simulink model "CrCtl_Governor"  (R2016b)
settings: configuration reference "CodeGenConfigSet" (kept outside this file)
values from neighbouring files (symbols this model uses):
  ACC_ZERO = fi(0,Acc_m_s2)    [init_CrCtl_Governor.m]
  CrCtl_facAcc2TrqCor_C = Calibration.Parameter    [init_CrCtl_Governor.m]
  CrCtl_facDecl2TrqCor_C = Calibration.Parameter    [init_CrCtl_Governor.m]
  CrCtl_facPT11_C = Calibration.Parameter    [init_CrCtl_Governor.m]
  CrCtl_facPT12_C = Calibration.Parameter    [init_CrCtl_Governor.m]
  CrCtl_facPT13_C = Calibration.Parameter    [init_CrCtl_Governor.m]
  CrCtl_facRmpSlpHiAcc_C = Calibration.Parameter    [init_CrCtl_Governor.m]
  CrCtl_facRmpSlpHiDecl_C = Calibration.Parameter    [init_CrCtl_Governor.m]
  CrCtl_facSlpConstRmpDwn_C = Calibration.Parameter    [init_CrCtl_Governor.m]
  CrCtl_facSlpConstRmpUp_C = Calibration.Parameter    [init_CrCtl_Governor.m]
  CrCtl_facSlpRmp1Sus_C = Calibration.Parameter    [init_CrCtl_Governor.m]
  CrCtl_facSlpRmp2Sus_C = Calibration.Parameter    [init_CrCtl_Governor.m]
  CrCtl_facTipDwnCor_CUR = Calibration.Parameter    [init_CrCtl_Governor.m]
  CrCtl_facTipDwnCor_CURX = Calibration.Parameter    [init_CrCtl_Governor.m]
  CrCtl_facTipUpCor_CUR = Calibration.Parameter    [init_CrCtl_Governor.m]
  CrCtl_facTipUpCor_CURX = Calibration.Parameter    [init_CrCtl_Governor.m]
  CrCtl_facTrqIncrSlpConstRmp_C = Calibration.Parameter    [init_CrCtl_Governor.m]
  CrCtl_facTrqIncrTimeConstRmp_C = Calibration.Parameter    [init_CrCtl_Governor.m]
  CrCtl_facTrqRedSlpConstRmp_C = Calibration.Parameter    [init_CrCtl_Governor.m]
  CrCtl_facTrqRedTimeConstRmp_C = Calibration.Parameter    [init_CrCtl_Governor.m]
  CrCtl_facTrqStrtAcc_C = Calibration.Parameter    [init_CrCtl_Governor.m]
  CrCtl_KiAcc1IWin_C = Calibration.Parameter    [init_CrCtl_Governor.m]
  CrCtl_KiAcc2IWin_C = Calibration.Parameter    [init_CrCtl_Governor.m]
  CrCtl_KiAcc3IWin_C = Calibration.Parameter    [init_CrCtl_Governor.m]
  CrCtl_KiCruise1IWin_C = Calibration.Parameter    [init_CrCtl_Governor.m]
  CrCtl_KiCruise2IWin_C = Calibration.Parameter    [init_CrCtl_Governor.m]
  CrCtl_KiCruise3IWin_C = Calibration.Parameter    [init_CrCtl_Governor.m]
  CrCtl_KiDecl1IWin_C = Calibration.Parameter    [init_CrCtl_Governor.m]
  CrCtl_KiDecl2IWin_C = Calibration.Parameter    [init_CrCtl_Governor.m]
  CrCtl_KiDecl3IWin_C = Calibration.Parameter    [init_CrCtl_Governor.m]
  CrCtl_KiNegAcc1IWin_C = Calibration.Parameter    [init_CrCtl_Governor.m]
  CrCtl_KiNegAcc2IWin_C = Calibration.Parameter    [init_CrCtl_Governor.m]
  CrCtl_KiNegAcc3IWin_C = Calibration.Parameter    [init_CrCtl_Governor.m]
  CrCtl_KiNegCruise1IWin_C = Calibration.Parameter    [init_CrCtl_Governor.m]
  CrCtl_KiNegCruise2IWin_C = Calibration.Parameter    [init_CrCtl_Governor.m]
  CrCtl_KiNegCruise3IWin_C = Calibration.Parameter    [init_CrCtl_Governor.m]
  CrCtl_KiNegDecl1IWin_C = Calibration.Parameter    [init_CrCtl_Governor.m]
  CrCtl_KiNegDecl2IWin_C = Calibration.Parameter    [init_CrCtl_Governor.m]
  CrCtl_KiNegDecl3IWin_C = Calibration.Parameter    [init_CrCtl_Governor.m]
  CrCtl_KiNegRes1IWin_C = Calibration.Parameter    [init_CrCtl_Governor.m]
  CrCtl_KiNegRes2IWin_C = Calibration.Parameter    [init_CrCtl_Governor.m]
  CrCtl_KiNegRes3IWin_C = Calibration.Parameter    [init_CrCtl_Governor.m]
  CrCtl_KiNegResCruise1IWin_C = Calibration.Parameter    [init_CrCtl_Governor.m]
  CrCtl_KiNegResCruise2IWin_C = Calibration.Parameter    [init_CrCtl_Governor.m]
  CrCtl_KiNegResCruise3IWin_C = Calibration.Parameter    [init_CrCtl_Governor.m]
  CrCtl_KiPosAcc1IWin_C = Calibration.Parameter    [init_CrCtl_Governor.m]
  CrCtl_KiPosAcc2IWin_C = Calibration.Parameter    [init_CrCtl_Governor.m]
  CrCtl_KiPosAcc3IWin_C = Calibration.Parameter    [init_CrCtl_Governor.m]
  CrCtl_KiPosCruise1IWin_C = Calibration.Parameter    [init_CrCtl_Governor.m]
  CrCtl_KiPosCruise2IWin_C = Calibration.Parameter    [init_CrCtl_Governor.m]
  CrCtl_KiPosCruise3IWin_C = Calibration.Parameter    [init_CrCtl_Governor.m]
  CrCtl_KiPosDecl1IWin_C = Calibration.Parameter    [init_CrCtl_Governor.m]
  CrCtl_KiPosDecl2IWin_C = Calibration.Parameter    [init_CrCtl_Governor.m]
  CrCtl_KiPosDecl3IWin_C = Calibration.Parameter    [init_CrCtl_Governor.m]
  CrCtl_KiPosRes1IWin_C = Calibration.Parameter    [init_CrCtl_Governor.m]
  CrCtl_KiPosRes3IWin_C = Calibration.Parameter    [init_CrCtl_Governor.m]
  CrCtl_KiPosResCruise1IWin_C = Calibration.Parameter    [init_CrCtl_Governor.m]
  CrCtl_KiPosResCruise2IWin_C = Calibration.Parameter    [init_CrCtl_Governor.m]
  CrCtl_KiPosResCruise3IWin_C = Calibration.Parameter    [init_CrCtl_Governor.m]
  CrCtl_KiRes1IWin_C = Calibration.Parameter    [init_CrCtl_Governor.m]
  CrCtl_KiRes2IWin_C = Calibration.Parameter    [init_CrCtl_Governor.m]
  CrCtl_KiRes3IWin_C = Calibration.Parameter    [init_CrCtl_Governor.m]
  CrCtl_KiResCruise1IWin_C = Calibration.Parameter    [init_CrCtl_Governor.m]
  CrCtl_KiResCruise2IWin_C = Calibration.Parameter    [init_CrCtl_Governor.m]
  CrCtl_KiResCruise3IWin_C = Calibration.Parameter    [init_CrCtl_Governor.m]
  CrCtl_KpAcc1PWin_C = Calibration.Parameter    [init_CrCtl_Governor.m]
  CrCtl_KpAcc2PWin_C = Calibration.Parameter    [init_CrCtl_Governor.m]
  CrCtl_KpAcc3PWin_C = Calibration.Parameter    [init_CrCtl_Governor.m]
  CrCtl_KpCruise1PWin_C = Calibration.Parameter    [init_CrCtl_Governor.m]
  CrCtl_KpCruise2PWin_C = Calibration.Parameter    [init_CrCtl_Governor.m]
  CrCtl_KpCruise3PWin_C = Calibration.Parameter    [init_CrCtl_Governor.m]
  CrCtl_KpDecl1PWin_C = Calibration.Parameter    [init_CrCtl_Governor.m]
  CrCtl_KpDecl2PWin_C = Calibration.Parameter    [init_CrCtl_Governor.m]
  CrCtl_KpDecl3PWin_C = Calibration.Parameter    [init_CrCtl_Governor.m]
  CrCtl_KpNegAcc1PWin_C = Calibration.Parameter    [init_CrCtl_Governor.m]
  CrCtl_KpNegAcc2PWin_C = Calibration.Parameter    [init_CrCtl_Governor.m]
  CrCtl_KpNegAcc3PWin_C = Calibration.Parameter    [init_CrCtl_Governor.m]
  CrCtl_KpNegCruise1PWin_C = Calibration.Parameter    [init_CrCtl_Governor.m]
  CrCtl_KpNegCruise2PWin_C = Calibration.Parameter    [init_CrCtl_Governor.m]
  CrCtl_KpNegCruise3PWin_C = Calibration.Parameter    [init_CrCtl_Governor.m]
  CrCtl_KpNegDecl1PWin_C = Calibration.Parameter    [init_CrCtl_Governor.m]
  CrCtl_KpNegDecl2PWin_C = Calibration.Parameter    [init_CrCtl_Governor.m]
  CrCtl_KpNegDecl3PWin_C = Calibration.Parameter    [init_CrCtl_Governor.m]
  CrCtl_KpNegRes1PWin_C = Calibration.Parameter    [init_CrCtl_Governor.m]
  CrCtl_KpNegRes2PWin_C = Calibration.Parameter    [init_CrCtl_Governor.m]
  CrCtl_KpNegRes3PWin_C = Calibration.Parameter    [init_CrCtl_Governor.m]
  CrCtl_KpNegResCruise1PWin_C = Calibration.Parameter    [init_CrCtl_Governor.m]
  CrCtl_KpNegResCruise2PWin_C = Calibration.Parameter    [init_CrCtl_Governor.m]
  CrCtl_KpNegResCruise3PWin_C = Calibration.Parameter    [init_CrCtl_Governor.m]
  CrCtl_KpPosAcc1PWin_C = Calibration.Parameter    [init_CrCtl_Governor.m]
  CrCtl_KpPosAcc2PWin_C = Calibration.Parameter    [init_CrCtl_Governor.m]
  CrCtl_KpPosAcc3PWin_C = Calibration.Parameter    [init_CrCtl_Governor.m]
  CrCtl_KpPosCruise1PWin_C = Calibration.Parameter    [init_CrCtl_Governor.m]
  CrCtl_KpPosCruise2PWin_C = Calibration.Parameter    [init_CrCtl_Governor.m]
  CrCtl_KpPosCruise3PWin_C = Calibration.Parameter    [init_CrCtl_Governor.m]
  CrCtl_KpPosDecl1PWin_C = Calibration.Parameter    [init_CrCtl_Governor.m]
  CrCtl_KpPosDecl2PWin_C = Calibration.Parameter    [init_CrCtl_Governor.m]
  CrCtl_KpPosDecl3PWin_C = Calibration.Parameter    [init_CrCtl_Governor.m]
  CrCtl_KpPosRes1PWin_C = Calibration.Parameter    [init_CrCtl_Governor.m]
  CrCtl_KpPosRes2PWin_C = Calibration.Parameter    [init_CrCtl_Governor.m]
  CrCtl_KpPosRes3PWin_C = Calibration.Parameter    [init_CrCtl_Governor.m]
  CrCtl_KpPosResCruise1PWin_C = Calibration.Parameter    [init_CrCtl_Governor.m]
  CrCtl_KpPosResCruise2PWin_C = Calibration.Parameter    [init_CrCtl_Governor.m]
  CrCtl_KpPosResCruise3PWin_C = Calibration.Parameter    [init_CrCtl_Governor.m]
  CrCtl_KpRes1PWin_C = Calibration.Parameter    [init_CrCtl_Governor.m]
  CrCtl_KpRes2PWin_C = Calibration.Parameter    [init_CrCtl_Governor.m]
  CrCtl_KpRes3PWin_C = Calibration.Parameter    [init_CrCtl_Governor.m]
  CrCtl_KpResCruise1PWin_C = Calibration.Parameter    [init_CrCtl_Governor.m]
  CrCtl_KpResCruise2PWin_C = Calibration.Parameter    [init_CrCtl_Governor.m]
  CrCtl_KpResCruise3PWin_C = Calibration.Parameter    [init_CrCtl_Governor.m]
  CrCtl_numParSelThres1_C = Calibration.Parameter    [init_CrCtl_Governor.m]
  CrCtl_numParSelThres2_C = Calibration.Parameter    [init_CrCtl_Governor.m]
  CrCtl_swtBrkMode_C = Calibration.Parameter    [init_CrCtl_Governor.m]
  CrCtl_swtILimWithP_C = Calibration.Parameter    [init_CrCtl_Governor.m]
  CrCtl_swtOvrRdeFrzInteg_C = Calibration.Parameter    [init_CrCtl_Governor.m]
  CrCtl_swtParSelHysBrk_C = Calibration.Parameter    [init_CrCtl_Governor.m]
  CrCtl_swtPT1EngBrk_C = Calibration.Parameter    [init_CrCtl_Governor.m]
  CrCtl_swtSusRmpInit_C = Calibration.Parameter    [init_CrCtl_Governor.m]
  CrCtl_swtSusRmpStp_C = Calibration.Parameter    [init_CrCtl_Governor.m]
  CrCtl_swtTipUpDwnGvnrStrtVal_C = Calibration.Parameter    [init_CrCtl_Governor.m]
  ... (+88 more)
undefined symbols (not defined in the file or in its folder): CrCtl_Governor_DT, CrCtl_stLck_conv, CrCtl_stOpFunc_conv, CrCtl_stShOff_conv, CrCtl_stSub_conv, CrCtl_stSuspRamp_conv, CruiseCtl_State_conv, EBrk_stPreSelMode_conv, WESDem_State_conv
libraries: CXLib x126, simulink x25
(part 4 of 6)

== system CrCtl_Governor/Cruise State/CRCTL_SUBGVNR/CrCtl_Suspend ==
  PT_trqWhlMinEng : Inport
  CrCtl_trqReqOld : Inport  Port=2
  AccPed_trqDes : Inport  Port=3
  CrCtl_trqLimAct : Inport  Port=4
  CrCtl_stSuspAct : Inport  Port=5
  Constant : Constant  Value=true
  Constant1 : Constant  Value=CrCtl_stSuspRamp_conv.CRCTL_SUSPENDENDRAMP
  Constant2 : Constant  Value=CrCtl_stSuspRamp_conv.CRCTL_SUSPENDRAMPDONE
  Constant3 : Constant  Value=CrCtl_stSuspRamp_conv.CRCTL_SUSPENDNOTACTIVE
  Constant4 : Constant  Value=CrCtl_stSuspRamp_conv.CRCTL_SUSPENDSTARTRAMP
  EdgeFalling : CXLib/EdgeFalling
  EdgeRising : CXLib/EdgeRising
  EdgeRising1 : CXLib/EdgeRising
  Logical Operator : Logic  Operator=NOT  AllPortsSameDT=off  OutDataTypeStr=boolean
  Subsystem : Subsystem
  Subsystem1 : Subsystem
  Switch{,1..3,5} (5 alike) : Switch  Criteria=u2 ~= 0
  Unit Delay : UnitDelay  SampleTime=-1
  CrCtl_stSuspRamp : Outport
  " CrCtl_trqReq" : Outport  Port=2
  wires:
  Subsystem/1(Out) -> Switch1/2, Subsystem1/5(In1)
  Subsystem/2(Out1) -> Switch5/1, Subsystem1/6(In2)
  PT_trqWhlMinEng/1 -> Subsystem/1(PT_trqWhlMinEng), Subsystem1/1(PT_trqWhlMinEng)
  CrCtl_trqReqOld/1 -> Subsystem/2(CrCtl_trqReqOld), Subsystem1/2(CrCtl_trqReqOld)
  CrCtl_trqLimAct/1 -> Subsystem1/4(CrCtl_trqLimAct)
  AccPed_trqDes/1 -> Subsystem1/3(AccPed_trqDes)
  Switch1/1 -> Switch/1
  Switch2/1 -> Switch/3
  Constant4/1 -> Switch1/1
  Constant2/1 -> Switch1/3
  Constant1/1 -> Switch2/1
  Constant3/1 -> Switch2/3
  Switch/1 -> CrCtl_stSuspRamp/1
  Subsystem1/1(Out1) -> Switch2/2
  Switch5/1 -> " CrCtl_trqReq"/1
  Subsystem1/2(Out2) -> Switch5/3
  Logical Operator/1 -> EdgeRising1/1
  EdgeRising/1 -> Subsystem/3(CrCtl_stSuspAct)
  EdgeRising1/1 -> Subsystem1/7(In3)
  CrCtl_stSuspAct/1 -> EdgeRising/1, EdgeFalling/1, Logical Operator/1, Subsystem/Enable, Switch/2, Switch5/2
  Constant/1 -> Switch3/1
  EdgeFalling/1 -> Switch3/2
  Switch3/1 -> Unit Delay/1, Subsystem1/Enable
  Unit Delay/1 -> Switch3/3

== system CrCtl_Governor/Cruise State/CRCTL_SUBGVNR/Governor ==
  CrCtl_trqLimAct : Inport
  CrCtl_trqMin : Inport  Port=2
  CrCtl_stGearRng_mp : Inport  Port=3
  CrCtl_vDesAct : Inport  Port=4
  stvHysEngBrkReq : Inport  Port=5
  GlbDa_vXFlt : Inport  Port=6
  stCrCtlOn : Inport  Port=7
  In1 : Inport  Port=8
  In2 : Inport  Port=9
  Enable : EnablePort
  Add1 : Sum  Inputs=+-
  Add2 : Sum  OutDataTypeStr=Trq_Nm
  Add3 : Sum  OutDataTypeStr=Trq_Nm
  Constant : Constant  Value=CrCtl_swtILimWithP_C
  Constant1 : Constant  Value=CrCtl_Governor_DT
  Constant2 : Constant  Value=1000  OutDataTypeStr=Inherit: Inherit via back propagation
  CrCtl_ARW : Subsystem
  I_S16 : CXLib/I_S16
  PT1 Filtered Torque : Subsystem
  P_S16 : CXLib/P_S16
  Parameter Selection for Ki : Subsystem
  Parameter Selection for Kp : Subsystem
  Product : Product  OutDataTypeStr=uint32
  Saturation_S16 : CXLib/Saturation_S16
  Switch : Switch  Criteria=u2 ~= 0
  Terminator : Terminator
  Unit Delay : UnitDelay  SampleTime=-1
  Unit Delay1 : UnitDelay  SampleTime=-1
  CrCtl_trqReq : Outport
  CrCtl_trqIWinOld_mp : Outport  Port=2  OutDataTypeStr=Trq_Nm
  CrCtl_trqReqPWin_mp : Outport  Port=3
  wires:
  CrCtl_vDesAct/1 -> Add1/1
  GlbDa_vXFlt/1 -> Add1/2
  Add1/1 -> PT1 Filtered Torque/2(vDiffCrCtl), I_S16/1, P_S16/1
  Add2/1 -> Add3/1
  PT1 Filtered Torque/1(CrCtl_trqDesvHys) -> Add3/2
  Add3/1 -> Saturation_S16/1
  CrCtl_trqMin/1 -> CrCtl_ARW/2(CrCtl_trqMin), Saturation_S16/2
  CrCtl_trqLimAct/1 -> CrCtl_ARW/3(CrCtl_trqLimAct), Saturation_S16/3
  Saturation_S16/2 -> Terminator/1
  Saturation_S16/1 -> CrCtl_trqReq/1
  Switch/1 -> CrCtl_ARW/5(CrCtl_trqReqIWin_mp), CrCtl_trqIWinOld_mp/1, Add2/2
  Constant/1 -> CrCtl_ARW/1(CrCtl_swtILimWithP_C)
  stvHysEngBrkReq/1 -> PT1 Filtered Torque/1(stvHysEngBrkReq)
  CrCtl_stGearRng_mp/1 -> Parameter Selection for Kp/1(CrCtl_stGearRng_mp), PT1 Filtered Torque/3(CrCtl_stGearRng_mp), Parameter Selection for Ki/1(CrCtl_stGearRng_mp)
  stCrCtlOn/1 -> PT1 Filtered Torque/4(stCrCtlOn)
  Parameter Selection for Kp/1(Out1) -> P_S16/2
  Parameter Selection for Kp/2(Out2) -> P_S16/3
  Parameter Selection for Kp/3(Out3) -> P_S16/4
  Parameter Selection for Kp/4(Out4) -> P_S16/5
  Parameter Selection for Kp/5(Out5) -> P_S16/6
  Parameter Selection for Ki/1(Out1) -> I_S16/3
  Parameter Selection for Ki/2(Out2) -> I_S16/4
  Parameter Selection for Ki/3(Out3) -> I_S16/5
  Parameter Selection for Ki/4(Out4) -> I_S16/6
  Parameter Selection for Ki/5(Out5) -> I_S16/7
  CrCtl_ARW/2(Limit) -> Unit Delay1/1
  CrCtl_ARW/1(CrCtl_stInit_mp) -> Unit Delay/1
  Product/1 -> I_S16/2
  Constant2/1 -> Product/2
  Constant1/1 -> Product/1
  I_S16/1 -> Switch/3
  Unit Delay1/1 -> Switch/1
  Unit Delay/1 -> Switch/2
  In1/1 -> I_S16/8
  In2/1 -> I_S16/9
  P_S16/1 -> CrCtl_trqReqPWin_mp/1, CrCtl_ARW/4(CrCtl_trqReqPWin_mp), Add2/1

== system CrCtl_Governor/Cruise State/CRCTL_SUBSTRTVAL/Parameter Selection for Kp ==
  CrCtl_stGearRng_mp : Inport
  Constant1 : Constant  Value=CrCtl_KpCruise2PWin_C
  Constant10 : Constant  Value=CrCtl_WinPosCruise1PWin_C
  Constant11 : Constant  Value=CrCtl_WinPosCruise2PWin_C
  Constant12 : Constant  Value=CrCtl_WinPosCruise2PWin_C
  Constant13 : Constant  Value=CrCtl_WinNegCruise1PWin_C
  Constant14 : Constant  Value=CrCtl_WinNegCruise2PWin_C
  Constant15 : Constant  Value=CrCtl_WinNegCruise3PWin_C
  Constant2 : Constant  Value=CrCtl_KpCruise3PWin_C
  Constant3 : Constant  Value=CrCtl_KpPosCruise1PWin_C
  Constant4 : Constant  Value=CrCtl_KpCruise1PWin_C
  Constant5 : Constant  Value=CrCtl_KpPosCruise2PWin_C
  Constant6 : Constant  Value=CrCtl_KpPosCruise3PWin_C
  Constant7 : Constant  Value=CrCtl_KpNegCruise1PWin_C
  Constant8 : Constant  Value=CrCtl_KpNegCruise2PWin_C
  Constant9 : Constant  Value=CrCtl_KpNegCruise3PWin_C
  Multiport Switch{,1..4} (5 alike) : MultiPortSwitch
  Out1 : Outport
  Out2 : Outport  Port=2
  Out3 : Outport  Port=3
  Out4 : Outport  Port=4
  Out5 : Outport  Port=5
  wires:
  CrCtl_stGearRng_mp/1 -> Multiport Switch4/1, Multiport Switch3/1, Multiport Switch2/1, Multiport Switch1/1, Multiport Switch/1
  Constant4/1 -> Multiport Switch/2
  Constant1/1 -> Multiport Switch/3
  Constant2/1 -> Multiport Switch/4
  Multiport Switch/1 -> Out1/1
  Constant3/1 -> Multiport Switch1/2
  Constant6/1 -> Multiport Switch1/4
  Constant5/1 -> Multiport Switch1/3
  Multiport Switch1/1 -> Out2/1
  Constant7/1 -> Multiport Switch2/2
  Constant9/1 -> Multiport Switch2/4
  Constant8/1 -> Multiport Switch2/3
  Constant10/1 -> Multiport Switch3/2
  Constant12/1 -> Multiport Switch3/4
  Constant11/1 -> Multiport Switch3/3
  Constant13/1 -> Multiport Switch4/2
  Constant15/1 -> Multiport Switch4/4
  Constant14/1 -> Multiport Switch4/3
  Multiport Switch2/1 -> Out3/1
  Multiport Switch3/1 -> Out4/1
  Multiport Switch4/1 -> Out5/1

== system CrCtl_Governor/Deceleration State/CRCTL_SUBRMP/CrCtl_OverRide ==
  CrCtl_trqLimAct : Inport
  CrCtl_trqMin : Inport  Port=2
  APP_r : Inport  Port=3
  AccPed_trqDes : Inport  Port=4
  CrCtl_vDes : Inport  Port=5
  GlbDa_vXFlt : Inport  Port=6
  CrCtl_trqReq : Inport  Port=7
  CrCtl_trqIWinOld_mp : Inport  Port=8
  Add : Sum
  Bit Clear : simulink/Logic and Bit Operations/Bit Clear  iBit=1
  Bit Clear7 : simulink/Logic and Bit Operations/Bit Clear  iBit=0
  Bit Set : simulink/Logic and Bit Operations/Bit Set  iBit=1
  Bit Set7 : simulink/Logic and Bit Operations/Bit Set  iBit=0
  Constant : Constant  Value=0
  Constant2 : Constant  Value=CrCtl_vCnclOverride_C
  Constant8 : Constant  Value=CrCtl_swtOvrRdeFrzInteg_C
  Logical Operator : Logic  AllPortsSameDT=off  OutDataTypeStr=boolean
  Logical Operator1 : Logic  AllPortsSameDT=off  OutDataTypeStr=boolean
  Relational Operator : RelationalOperator  Operator=>  OutDataTypeStr=boolean  RndMeth=Simplest
  Relational Operator1 : RelationalOperator  Operator=>  OutDataTypeStr=boolean  RndMeth=Simplest
  Relational Operator2 : RelationalOperator  Operator=<=  OutDataTypeStr=boolean  RndMeth=Simplest
  Relational Operator3 : RelationalOperator  Operator=<  OutDataTypeStr=boolean  RndMeth=Simplest
  Saturation_S16 : CXLib/Saturation_S16
  Switch : Switch  Criteria=u2 ~= 0
  Switch7 : Switch  Criteria=u2 ~= 0
  Switch8 : Switch  Criteria=u2 ~= 0
  Terminator1 : Terminator
  Unit Delay : UnitDelay  SampleTime=-1
  CrCtl_stIWin_mp : Outport
  CrCtl_trqReqIWin_mp : Outport  Port=2
  wires:
  APP_r/1 -> Relational Operator/1
  Constant/1 -> Relational Operator/2
  AccPed_trqDes/1 -> Relational Operator1/1, Relational Operator2/1
  Relational Operator/1 -> Logical Operator/1
  Relational Operator1/1 -> Logical Operator/2
  Logical Operator/1 -> Switch/2
  Relational Operator2/1 -> Logical Operator1/1
  Relational Operator3/1 -> Logical Operator1/2
  GlbDa_vXFlt/1 -> Relational Operator3/1
  CrCtl_vDes/1 -> Add/1
  Add/1 -> Relational Operator3/2
  Constant2/1 -> Add/2
  CrCtl_trqLimAct/1 -> Saturation_S16/3
  CrCtl_trqMin/1 -> Saturation_S16/2
  Bit Set/1 -> Switch/1
  Bit Clear/1 -> Switch/3
  Switch/1 -> Bit Clear7/1, Bit Set7/1
  Constant8/1 -> Switch7/2
  Bit Set7/1 -> Switch7/1
  Bit Clear7/1 -> Switch7/3
  Switch7/1 -> CrCtl_stIWin_mp/1, Unit Delay/1
  Unit Delay/1 -> Bit Set/1, Bit Clear/1
  CrCtl_trqReq/1 -> Saturation_S16/1
  Saturation_S16/1 -> Switch8/3, Relational Operator2/2, Relational Operator1/2
  Saturation_S16/2 -> Terminator1/1
  Logical Operator1/1 -> Switch8/2
  CrCtl_trqIWinOld_mp/1 -> Switch8/1
  Switch8/1 -> CrCtl_trqReqIWin_mp/1

== system CrCtl_Governor/Deceleration State/CRCTL_SUBRMP/CrCtl_Suspend ==
  PT_trqWhlMinEng : Inport
  CrCtl_trqReqOld : Inport  Port=2
  AccPed_trqDes : Inport  Port=3
  CrCtl_trqLimAct : Inport  Port=4
  CrCtl_stSuspAct : Inport  Port=5
  Constant : Constant  Value=true
  Constant1 : Constant  Value=CrCtl_stSuspRamp_conv.CRCTL_SUSPENDENDRAMP
  Constant2 : Constant  Value=CrCtl_stSuspRamp_conv.CRCTL_SUSPENDRAMPDONE
  Constant3 : Constant  Value=CrCtl_stSuspRamp_conv.CRCTL_SUSPENDNOTACTIVE
  Constant4 : Constant  Value=CrCtl_stSuspRamp_conv.CRCTL_SUSPENDSTARTRAMP
  EdgeFalling : CXLib/EdgeFalling
  EdgeRising : CXLib/EdgeRising
  EdgeRising1 : CXLib/EdgeRising
  Logical Operator : Logic  Operator=NOT  AllPortsSameDT=off  OutDataTypeStr=boolean
  Subsystem : Subsystem
  Subsystem1 : Subsystem
  Switch{,1..3,5} (5 alike) : Switch  Criteria=u2 ~= 0
  Unit Delay : UnitDelay  SampleTime=-1
  CrCtl_stSuspRamp : Outport
  " CrCtl_trqReq" : Outport  Port=2
  wires:
  Subsystem/1(Out) -> Switch1/2, Subsystem1/5(In1)
  Subsystem/2(Out1) -> Switch5/1, Subsystem1/6(In2)
  PT_trqWhlMinEng/1 -> Subsystem/1(PT_trqWhlMinEng), Subsystem1/1(PT_trqWhlMinEng)
  CrCtl_trqReqOld/1 -> Subsystem/2(CrCtl_trqReqOld), Subsystem1/2(CrCtl_trqReqOld)
  CrCtl_trqLimAct/1 -> Subsystem1/4(CrCtl_trqLimAct)
  AccPed_trqDes/1 -> Subsystem1/3(AccPed_trqDes)
  Switch1/1 -> Switch/1
  Switch2/1 -> Switch/3
  Constant4/1 -> Switch1/1
  Constant2/1 -> Switch1/3
  Constant1/1 -> Switch2/1
  Constant3/1 -> Switch2/3
  Switch/1 -> CrCtl_stSuspRamp/1
  Subsystem1/1(Out1) -> Switch2/2
  Switch5/1 -> " CrCtl_trqReq"/1
  Subsystem1/2(Out2) -> Switch5/3
  Logical Operator/1 -> EdgeRising1/1
  EdgeRising/1 -> Subsystem/3(CrCtl_stSuspAct)
  EdgeRising1/1 -> Subsystem1/7(In3)
  CrCtl_stSuspAct/1 -> EdgeRising/1, EdgeFalling/1, Logical Operator/1, Subsystem/Enable, Switch/2, Switch5/2
  Constant/1 -> Switch3/1
  EdgeFalling/1 -> Switch3/2
  Switch3/1 -> Unit Delay/1, Subsystem1/Enable
  Unit Delay/1 -> Switch3/3

== system CrCtl_Governor/Deceleration State/CRCTL_SUBRMP/Governor ==
  CrCtl_trqLimAct : Inport
  CrCtl_trqMin : Inport  Port=2
  CrCtl_stGearRng_mp : Inport  Port=3
  CrCtl_vDesAct : Inport  Port=4
  stvHysEngBrkReq : Inport  Port=5
  GlbDa_vXFlt : Inport  Port=6
  stCrCtlOn : Inport  Port=7
  In1 : Inport  Port=8
  In2 : Inport  Port=9
  Enable : EnablePort
  Add1 : Sum  Inputs=+-
  Add2 : Sum  OutDataTypeStr=Trq_Nm
  Add3 : Sum  OutDataTypeStr=Trq_Nm
  Constant : Constant  Value=CrCtl_swtILimWithP_C
  Constant1 : Constant  Value=CrCtl_Governor_DT
  Constant2 : Constant  Value=1000  OutDataTypeStr=Inherit: Inherit via back propagation
  CrCtl_ARW : Subsystem
  I_S16 : CXLib/I_S16
  PT1 Filtered Torque : Subsystem
  P_S16 : CXLib/P_S16
  Parameter Selection for Ki : Subsystem
  Parameter Selection for Kp : Subsystem
  Product : Product  OutDataTypeStr=uint32
  Saturation_S16 : CXLib/Saturation_S16
  Switch : Switch  Criteria=u2 ~= 0
  Terminator : Terminator
  Unit Delay : UnitDelay  SampleTime=-1
  Unit Delay1 : UnitDelay  SampleTime=-1
  CrCtl_trqReq : Outport
  CrCtl_trqIWinOld_mp : Outport  Port=2  OutDataTypeStr=Trq_Nm
  CrCtl_trqReqPWin_mp : Outport  Port=3
  wires:
  CrCtl_vDesAct/1 -> Add1/1
  GlbDa_vXFlt/1 -> Add1/2
  Add1/1 -> PT1 Filtered Torque/2(vDiffCrCtl), I_S16/1, P_S16/1
  Add2/1 -> Add3/1
  PT1 Filtered Torque/1(CrCtl_trqDesvHys) -> Add3/2
  Add3/1 -> Saturation_S16/1
  CrCtl_trqMin/1 -> CrCtl_ARW/2(CrCtl_trqMin), Saturation_S16/2
  CrCtl_trqLimAct/1 -> CrCtl_ARW/3(CrCtl_trqLimAct), Saturation_S16/3
  Saturation_S16/2 -> Terminator/1
  Saturation_S16/1 -> CrCtl_trqReq/1
  Switch/1 -> CrCtl_ARW/5(CrCtl_trqReqIWin_mp), CrCtl_trqIWinOld_mp/1, Add2/2
  Constant/1 -> CrCtl_ARW/1(CrCtl_swtILimWithP_C)
  stvHysEngBrkReq/1 -> PT1 Filtered Torque/1(stvHysEngBrkReq)
  CrCtl_stGearRng_mp/1 -> Parameter Selection for Kp/1(CrCtl_stGearRng_mp), Parameter Selection for Ki/1(CrCtl_stGearRng_mp), PT1 Filtered Torque/3(CrCtl_stGearRng_mp)
  stCrCtlOn/1 -> PT1 Filtered Torque/4(stCrCtlOn)
  Parameter Selection for Kp/1(Out1) -> P_S16/2
  Parameter Selection for Kp/2(Out2) -> P_S16/3
  Parameter Selection for Kp/3(Out3) -> P_S16/4
  Parameter Selection for Kp/4(Out4) -> P_S16/5
  Parameter Selection for Kp/5(Out5) -> P_S16/6
  Parameter Selection for Ki/1(Out1) -> I_S16/3
  Parameter Selection for Ki/2(Out2) -> I_S16/4
  Parameter Selection for Ki/3(Out3) -> I_S16/5
  Parameter Selection for Ki/4(Out4) -> I_S16/6
  Parameter Selection for Ki/5(Out5) -> I_S16/7
  CrCtl_ARW/2(Limit) -> Unit Delay1/1
  CrCtl_ARW/1(CrCtl_stInit_mp) -> Unit Delay/1
  Product/1 -> I_S16/2
  Constant2/1 -> Product/2
  Constant1/1 -> Product/1
  P_S16/1 -> CrCtl_trqReqPWin_mp/1, CrCtl_ARW/4(CrCtl_trqReqPWin_mp), Add2/1
  In1/1 -> I_S16/8
  In2/1 -> I_S16/9
  I_S16/1 -> Switch/3
  Unit Delay1/1 -> Switch/1
  Unit Delay/1 -> Switch/2

== system CrCtl_Governor/OFF State/CRCTL_SUBRMP/Immediate Shut off demanded ==
  PT_trqWhlMinEng : Inport
  Enable : EnablePort
  CrCtl_trqReq : Outport
  wires:
  PT_trqWhlMinEng/1 -> CrCtl_trqReq/1

== system CrCtl_Governor/OFF State/CRCTL_SUBRMP/Shut off by Slope Constant Ramp demanded ==
  PT_trqWhlMinEng : Inport
  CrCtl_trqReqOld : Inport  Port=2
  In1 : Inport  Port=3
  Enable : EnablePort
  Add : Sum
  Add1 : Sum  Inputs=+-
  Add2 : Sum  Inputs=+-
  Add3 : Sum  Inputs=+-
  Constant : Constant  Value=CrCtl_facTrqIncrSlpConstRmp_C
  Constant1 : Constant  Value=CrCtl_Governor_DT
  Constant2 : Constant  Value=CrCtl_facTrqRedSlpConstRmp_C
  Constant3 : Constant  Value=CrCtl_facSlpConstRmpUp_C
  Constant4 : Constant  Value=CrCtl_Governor_DT
  Constant5 : Constant  Value=CrCtl_facSlpConstRmpDwn_C
  Product : Product  OutDataTypeStr=Trq_Nm
  Product1 : Product  OutDataTypeStr=Trq_Nm
  RAMP_S16 : CXLib/RAMP_S16
  Relational Operator : RelationalOperator  Operator=>  OutDataTypeStr=boolean  RndMeth=Simplest
  Switch : Switch  Criteria=u2 ~= 0
  s2dt : CXLib/s2dt
  s2dt1 : CXLib/s2dt
  CrCtl_trqReq : Outport
  wires:
  s2dt/1 -> RAMP_S16/2
  Constant3/1 -> s2dt/1
  Constant4/1 -> s2dt/2
  Switch/1 -> RAMP_S16/5
  Constant1/1 -> s2dt1/2
  PT_trqWhlMinEng/1 -> RAMP_S16/1, Relational Operator/2, Add2/2, Add1/1
  Relational Operator/1 -> Switch/2
  CrCtl_trqReqOld/1 -> Add/1, Relational Operator/1, Add1/2, Add3/1, Add2/1
  Add1/1 -> Product/1
  Add2/1 -> Product1/2
  Constant/1 -> Product/2
  Constant2/1 -> Product1/1
  Product/1 -> Add/2
  Product1/1 -> Add3/2
  Add/1 -> Switch/3
  Add3/1 -> Switch/1
  s2dt1/1 -> RAMP_S16/3
  Constant5/1 -> s2dt1/1
  In1/1 -> RAMP_S16/4
  RAMP_S16/1 -> CrCtl_trqReq/1

== system CrCtl_Governor/OFF State/CRCTL_SUBRMP/Shut off by Time Constant Ramp demanded ==
  PT_trqWhlMinEng : Inport
  CrCtl_trqReqOld : Inport  Port=2
  In1 : Inport  Port=3
  Enable : EnablePort
  Abs : Abs
  Add : Sum
  Add1 : Sum  Inputs=+-
  Add2 : Sum  Inputs=+-
  Add3 : Sum  Inputs=+-
  Constant : Constant  Value=CrCtl_facTrqIncrTimeConstRmp_C
  Constant1 : Constant  Value=CrCtl_Governor_DT
  Constant2 : Constant  Value=CrCtl_facTrqRedTimeConstRmp_C
  Constant4 : Constant  Value=CrCtl_Governor_DT
  Constant6 : Constant  Value=CrCtl_tiShDwnTimeCnstRmp_C
  Divide : Product  Inputs=*/  OutDataTypeStr=Inherit: Inherit via back propagation
  Product : Product  OutDataTypeStr=Trq_Nm
  Product1 : Product  OutDataTypeStr=Trq_Nm
  RAMP_S16 : CXLib/RAMP_S16
  Relational Operator : RelationalOperator  Operator=>  OutDataTypeStr=boolean  RndMeth=Simplest
  Switch : Switch  Criteria=u2 ~= 0
  s2dt : CXLib/s2dt
  s2dt1 : CXLib/s2dt
  CrCtl_trqReq : Outport
  wires:
  PT_trqWhlMinEng/1 -> RAMP_S16/1, Add2/2, Add1/1, Relational Operator/2
  Relational Operator/1 -> Switch/2
  CrCtl_trqReqOld/1 -> Add2/1, Add3/1, Add1/2, Add/1, Relational Operator/1
  Add1/1 -> Abs/1, Product/1
  Add2/1 -> Product1/2
  Constant/1 -> Product/2
  Constant2/1 -> Product1/1
  Product/1 -> Add/2
  Product1/1 -> Add3/2
  Add/1 -> Switch/3
  Add3/1 -> Switch/1
  Divide/1 -> s2dt/1, s2dt1/1  "CrCtl_facShDwnTimeCnstRmp_mp"
  Constant4/1 -> s2dt/2
  Constant1/1 -> s2dt1/2
  s2dt1/1 -> RAMP_S16/3
  RAMP_S16/1 -> CrCtl_trqReq/1
  Abs/1 -> Divide/1
  Constant6/1 -> Divide/2
  In1/1 -> RAMP_S16/4
  Switch/1 -> RAMP_S16/5
  s2dt/1 -> RAMP_S16/2

== system CrCtl_Governor/Resume From Above/CRCTL_SUBRMP/CrCtl_OverRide ==
  CrCtl_trqLimAct : Inport
  CrCtl_trqMin : Inport  Port=2
  APP_r : Inport  Port=3
  AccPed_trqDes : Inport  Port=4
  CrCtl_vDes : Inport  Port=5
  GlbDa_vXFlt : Inport  Port=6
  CrCtl_trqReq : Inport  Port=7
  CrCtl_trqIWinOld_mp : Inport  Port=8
  Add : Sum
  Bit Clear : simulink/Logic and Bit Operations/Bit Clear  iBit=1
  Bit Clear7 : simulink/Logic and Bit Operations/Bit Clear  iBit=0
  Bit Set : simulink/Logic and Bit Operations/Bit Set  iBit=1
  Bit Set7 : simulink/Logic and Bit Operations/Bit Set  iBit=0
  Constant : Constant  Value=0
  Constant2 : Constant  Value=CrCtl_vCnclOverride_C
  Constant8 : Constant  Value=CrCtl_swtOvrRdeFrzInteg_C
  Logical Operator : Logic  AllPortsSameDT=off  OutDataTypeStr=boolean
  Logical Operator1 : Logic  AllPortsSameDT=off  OutDataTypeStr=boolean
  Relational Operator : RelationalOperator  Operator=>  OutDataTypeStr=boolean  RndMeth=Simplest
  Relational Operator1 : RelationalOperator  Operator=>  OutDataTypeStr=boolean  RndMeth=Simplest
  Relational Operator2 : RelationalOperator  Operator=<=  OutDataTypeStr=boolean  RndMeth=Simplest
  Relational Operator3 : RelationalOperator  Operator=<  OutDataTypeStr=boolean  RndMeth=Simplest
  Saturation_S16 : CXLib/Saturation_S16
  Switch : Switch  Criteria=u2 ~= 0
  Switch7 : Switch  Criteria=u2 ~= 0
  Switch8 : Switch  Criteria=u2 ~= 0
  Terminator1 : Terminator
  Unit Delay : UnitDelay  SampleTime=-1
  CrCtl_stIWin_mp : Outport
  CrCtl_trqReqIWin_mp : Outport  Port=2
  wires:
  APP_r/1 -> Relational Operator/1
  Constant/1 -> Relational Operator/2
  AccPed_trqDes/1 -> Relational Operator1/1, Relational Operator2/1
  Relational Operator/1 -> Logical Operator/1
  Relational Operator1/1 -> Logical Operator/2
  Logical Operator/1 -> Switch/2
  Relational Operator2/1 -> Logical Operator1/1
  Relational Operator3/1 -> Logical Operator1/2
  GlbDa_vXFlt/1 -> Relational Operator3/1
  CrCtl_vDes/1 -> Add/1
  Add/1 -> Relational Operator3/2
  Constant2/1 -> Add/2
  CrCtl_trqLimAct/1 -> Saturation_S16/3
  CrCtl_trqMin/1 -> Saturation_S16/2
  Bit Set/1 -> Switch/1
  Bit Clear/1 -> Switch/3
  Switch/1 -> Bit Clear7/1, Bit Set7/1
  Constant8/1 -> Switch7/2
  Bit Set7/1 -> Switch7/1
  Bit Clear7/1 -> Switch7/3
  Switch7/1 -> CrCtl_stIWin_mp/1, Unit Delay/1
  Unit Delay/1 -> Bit Set/1, Bit Clear/1
  CrCtl_trqReq/1 -> Saturation_S16/1
  Saturation_S16/1 -> Switch8/3, Relational Operator2/2, Relational Operator1/2
  Saturation_S16/2 -> Terminator1/1
  Logical Operator1/1 -> Switch8/2
  CrCtl_trqIWinOld_mp/1 -> Switch8/1
  Switch8/1 -> CrCtl_trqReqIWin_mp/1

== system CrCtl_Governor/Resume From Above/CRCTL_SUBRMP/CrCtl_Suspend ==
  PT_trqWhlMinEng : Inport
  CrCtl_trqReqOld : Inport  Port=2
  AccPed_trqDes : Inport  Port=3
  CrCtl_trqLimAct : Inport  Port=4
  CrCtl_stSuspAct : Inport  Port=5
  Constant : Constant  Value=true
  Constant1 : Constant  Value=CrCtl_stSuspRamp_conv.CRCTL_SUSPENDENDRAMP
  Constant2 : Constant  Value=CrCtl_stSuspRamp_conv.CRCTL_SUSPENDRAMPDONE
  Constant3 : Constant  Value=CrCtl_stSuspRamp_conv.CRCTL_SUSPENDNOTACTIVE
  Constant4 : Constant  Value=CrCtl_stSuspRamp_conv.CRCTL_SUSPENDSTARTRAMP
  EdgeFalling : CXLib/EdgeFalling
  EdgeRising : CXLib/EdgeRising
  EdgeRising1 : CXLib/EdgeRising
  Logical Operator : Logic  Operator=NOT  AllPortsSameDT=off  OutDataTypeStr=boolean
  Subsystem : Subsystem
  Subsystem1 : Subsystem
  Switch{,1..3,5} (5 alike) : Switch  Criteria=u2 ~= 0
  Unit Delay : UnitDelay  SampleTime=-1
  CrCtl_stSuspRamp : Outport
  " CrCtl_trqReq" : Outport  Port=2
  wires:
  Subsystem/1(Out) -> Switch1/2, Subsystem1/5(In1)
  Subsystem/2(Out1) -> Switch5/1, Subsystem1/6(In2)
  PT_trqWhlMinEng/1 -> Subsystem/1(PT_trqWhlMinEng), Subsystem1/1(PT_trqWhlMinEng)
  CrCtl_trqReqOld/1 -> Subsystem/2(CrCtl_trqReqOld), Subsystem1/2(CrCtl_trqReqOld)
  CrCtl_trqLimAct/1 -> Subsystem1/4(CrCtl_trqLimAct)
  AccPed_trqDes/1 -> Subsystem1/3(AccPed_trqDes)
  Switch1/1 -> Switch/1
  Switch2/1 -> Switch/3
  Constant4/1 -> Switch1/1
  Constant2/1 -> Switch1/3
  Constant1/1 -> Switch2/1
  Constant3/1 -> Switch2/3
  Switch/1 -> CrCtl_stSuspRamp/1
  Subsystem1/1(Out1) -> Switch2/2
  Switch5/1 -> " CrCtl_trqReq"/1
  Subsystem1/2(Out2) -> Switch5/3
  Logical Operator/1 -> EdgeRising1/1
  EdgeRising/1 -> Subsystem/3(CrCtl_stSuspAct)
  EdgeRising1/1 -> Subsystem1/7(In3)
  CrCtl_stSuspAct/1 -> EdgeRising/1, EdgeFalling/1, Logical Operator/1, Subsystem/Enable, Switch/2, Switch5/2
  Constant/1 -> Switch3/1
  EdgeFalling/1 -> Switch3/2
  Switch3/1 -> Unit Delay/1, Subsystem1/Enable
  Unit Delay/1 -> Switch3/3

== system CrCtl_Governor/Resume From Above/CRCTL_SUBRMP/Governor ==
  CrCtl_trqLimAct : Inport
  CrCtl_trqMin : Inport  Port=2
  CrCtl_stGearRng_mp : Inport  Port=3
  CrCtl_vDesAct : Inport  Port=4
  stvHysEngBrkReq : Inport  Port=5
  GlbDa_vXFlt : Inport  Port=6
  stCrCtlOn : Inport  Port=7
  In1 : Inport  Port=8
  In2 : Inport  Port=9
  Enable : EnablePort
  Add1 : Sum  Inputs=+-
  Add2 : Sum  OutDataTypeStr=Trq_Nm
  Add3 : Sum  OutDataTypeStr=Trq_Nm
  Constant : Constant  Value=CrCtl_swtILimWithP_C
  Constant1 : Constant  Value=CrCtl_Governor_DT
  Constant2 : Constant  Value=1000  OutDataTypeStr=Inherit: Inherit via back propagation
  CrCtl_ARW : Subsystem
  I_S16 : CXLib/I_S16
  PT1 Filtered Torque : Subsystem
  P_S16 : CXLib/P_S16
  Parameter Selection for Ki : Subsystem
  Parameter Selection for Kp : Subsystem
  Product : Product  OutDataTypeStr=uint32
  Saturation_S16 : CXLib/Saturation_S16
  Switch : Switch  Criteria=u2 ~= 0
  Terminator : Terminator
  Unit Delay : UnitDelay  SampleTime=-1
  Unit Delay1 : UnitDelay  SampleTime=-1
  CrCtl_trqReq : Outport
  CrCtl_trqIWinOld_mp : Outport  Port=2  OutDataTypeStr=Trq_Nm
  CrCtl_trqReqPWin_mp : Outport  Port=3
  wires:
  CrCtl_vDesAct/1 -> Add1/1
  GlbDa_vXFlt/1 -> Add1/2
  Add1/1 -> PT1 Filtered Torque/2(vDiffCrCtl), I_S16/1, P_S16/1
  Add2/1 -> Add3/1
  PT1 Filtered Torque/1(CrCtl_trqDesvHys) -> Add3/2
  Add3/1 -> Saturation_S16/1
  CrCtl_trqMin/1 -> CrCtl_ARW/2(CrCtl_trqMin), Saturation_S16/2
  CrCtl_trqLimAct/1 -> CrCtl_ARW/3(CrCtl_trqLimAct), Saturation_S16/3
  Saturation_S16/2 -> Terminator/1
  Saturation_S16/1 -> CrCtl_trqReq/1
  Switch/1 -> Add2/2, CrCtl_trqIWinOld_mp/1, CrCtl_ARW/5(CrCtl_trqReqIWin_mp)
  Constant/1 -> CrCtl_ARW/1(CrCtl_swtILimWithP_C)
  stvHysEngBrkReq/1 -> PT1 Filtered Torque/1(stvHysEngBrkReq)
  CrCtl_stGearRng_mp/1 -> Parameter Selection for Kp/1(CrCtl_stGearRng_mp), Parameter Selection for Ki/1(CrCtl_stGearRng_mp), PT1 Filtered Torque/3(CrCtl_stGearRng_mp)
  stCrCtlOn/1 -> PT1 Filtered Torque/4(stCrCtlOn)
  Parameter Selection for Kp/1(Out1) -> P_S16/2
  Parameter Selection for Kp/2(Out2) -> P_S16/3
  Parameter Selection for Kp/3(Out3) -> P_S16/4
  Parameter Selection for Kp/4(Out4) -> P_S16/5
  Parameter Selection for Kp/5(Out5) -> P_S16/6
  Parameter Selection for Ki/1(Out1) -> I_S16/3
  Parameter Selection for Ki/2(Out2) -> I_S16/4
  Parameter Selection for Ki/3(Out3) -> I_S16/5
  Parameter Selection for Ki/4(Out4) -> I_S16/6
  Parameter Selection for Ki/5(Out5) -> I_S16/7
  CrCtl_ARW/2(Limit) -> Unit Delay1/1
  CrCtl_ARW/1(CrCtl_stInit_mp) -> Unit Delay/1
  Product/1 -> I_S16/2
  Constant2/1 -> Product/2
  Constant1/1 -> Product/1
  P_S16/1 -> CrCtl_trqReqPWin_mp/1, CrCtl_ARW/4(CrCtl_trqReqPWin_mp), Add2/1
  I_S16/1 -> Switch/3
  In1/1 -> I_S16/8
  In2/1 -> I_S16/9
  Unit Delay1/1 -> Switch/1
  Unit Delay/1 -> Switch/2

== system CrCtl_Governor/Resume From Above/CRCTL_SUBSTRTVAL/Parameter Selection for Kp ==
  CrCtl_stGearRng_mp : Inport
  Constant1 : Constant  Value=CrCtl_KpRes2PWin_C
  Constant10 : Constant  Value=CrCtl_WinPosRes1PWin_C
  Constant11 : Constant  Value=CrCtl_WinPosRes2PWin_C
  Constant12 : Constant  Value=CrCtl_WinPosRes3PWin_C
  Constant13 : Constant  Value=CrCtl_WinNegRes1PWin_C
  Constant14 : Constant  Value=CrCtl_WinNegRes2PWin_C
  Constant15 : Constant  Value=CrCtl_WinNegRes3PWin_C
  Constant2 : Constant  Value=CrCtl_KpRes3PWin_C
  Constant3 : Constant  Value=CrCtl_KpPosRes1PWin_C
  Constant4 : Constant  Value=CrCtl_KpRes1PWin_C
  Constant5 : Constant  Value=CrCtl_KpPosRes2PWin_C
  Constant6 : Constant  Value=CrCtl_KpPosRes3PWin_C
  Constant7 : Constant  Value=CrCtl_KpNegRes1PWin_C
  Constant8 : Constant  Value=CrCtl_KpNegRes2PWin_C
  Constant9 : Constant  Value=CrCtl_KpNegRes3PWin_C
  Multiport Switch{,1..4} (5 alike) : MultiPortSwitch
  Out1 : Outport
  Out2 : Outport  Port=2
  Out3 : Outport  Port=3
  Out4 : Outport  Port=4
  Out5 : Outport  Port=5
  wires:
  CrCtl_stGearRng_mp/1 -> Multiport Switch4/1, Multiport Switch3/1, Multiport Switch2/1, Multiport Switch1/1, Multiport Switch/1
  Constant4/1 -> Multiport Switch/2
  Constant1/1 -> Multiport Switch/3
  Constant2/1 -> Multiport Switch/4
  Multiport Switch/1 -> Out1/1
  Constant3/1 -> Multiport Switch1/2
  Constant6/1 -> Multiport Switch1/4
  Constant5/1 -> Multiport Switch1/3
  Multiport Switch1/1 -> Out2/1
  Constant7/1 -> Multiport Switch2/2
  Constant9/1 -> Multiport Switch2/4
  Constant8/1 -> Multiport Switch2/3
  Constant10/1 -> Multiport Switch3/2
  Constant12/1 -> Multiport Switch3/4
  Constant11/1 -> Multiport Switch3/3
  Constant13/1 -> Multiport Switch4/2
  Constant15/1 -> Multiport Switch4/4
  Constant14/1 -> Multiport Switch4/3
  Multiport Switch2/1 -> Out3/1
  Multiport Switch3/1 -> Out4/1
  Multiport Switch4/1 -> Out5/1

== system CrCtl_Governor/Resume From Below/CRCTL_SUBPRECRUISE/CrCtl_OverRide ==
  CrCtl_trqLimAct : Inport
  CrCtl_trqMin : Inport  Port=2
  APP_r : Inport  Port=3
  AccPed_trqDes : Inport  Port=4
  CrCtl_vDes : Inport  Port=5
  GlbDa_vXFlt : Inport  Port=6
  CrCtl_trqReq : Inport  Port=7
  CrCtl_trqIWinOld_mp : Inport  Port=8
  Add : Sum
  Bit Clear : simulink/Logic and Bit Operations/Bit Clear  iBit=1
  Bit Clear7 : simulink/Logic and Bit Operations/Bit Clear  iBit=0
  Bit Set : simulink/Logic and Bit Operations/Bit Set  iBit=1
  Bit Set7 : simulink/Logic and Bit Operations/Bit Set  iBit=0
  Constant : Constant  Value=0
  Constant2 : Constant  Value=CrCtl_vCnclOverride_C
  Constant8 : Constant  Value=CrCtl_swtOvrRdeFrzInteg_C
  Logical Operator : Logic  AllPortsSameDT=off  OutDataTypeStr=boolean
  Logical Operator1 : Logic  AllPortsSameDT=off  OutDataTypeStr=boolean
  Relational Operator : RelationalOperator  Operator=>  OutDataTypeStr=boolean  RndMeth=Simplest
  Relational Operator1 : RelationalOperator  Operator=>  OutDataTypeStr=boolean  RndMeth=Simplest
  Relational Operator2 : RelationalOperator  Operator=<=  OutDataTypeStr=boolean  RndMeth=Simplest
  Relational Operator3 : RelationalOperator  Operator=<  OutDataTypeStr=boolean  RndMeth=Simplest
  Saturation_S16 : CXLib/Saturation_S16
  Switch : Switch  Criteria=u2 ~= 0
  Switch7 : Switch  Criteria=u2 ~= 0
  Switch8 : Switch  Criteria=u2 ~= 0
  Terminator1 : Terminator
  Unit Delay : UnitDelay  SampleTime=-1
  CrCtl_stIWin_mp : Outport
  CrCtl_trqReqIWin_mp : Outport  Port=2
  wires:
  APP_r/1 -> Relational Operator/1
  Constant/1 -> Relational Operator/2
  AccPed_trqDes/1 -> Relational Operator1/1, Relational Operator2/1
  Relational Operator/1 -> Logical Operator/1
  Relational Operator1/1 -> Logical Operator/2
  Logical Operator/1 -> Switch/2
  Relational Operator2/1 -> Logical Operator1/1
  Relational Operator3/1 -> Logical Operator1/2
  GlbDa_vXFlt/1 -> Relational Operator3/1
  CrCtl_vDes/1 -> Add/1
  Add/1 -> Relational Operator3/2
  Constant2/1 -> Add/2
  CrCtl_trqLimAct/1 -> Saturation_S16/3
  CrCtl_trqMin/1 -> Saturation_S16/2
  Bit Set/1 -> Switch/1
  Bit Clear/1 -> Switch/3
  Switch/1 -> Bit Clear7/1, Bit Set7/1
  Constant8/1 -> Switch7/2
  Bit Set7/1 -> Switch7/1
  Bit Clear7/1 -> Switch7/3
  Switch7/1 -> CrCtl_stIWin_mp/1, Unit Delay/1
  Unit Delay/1 -> Bit Set/1, Bit Clear/1
  CrCtl_trqReq/1 -> Saturation_S16/1
  Saturation_S16/1 -> Switch8/3, Relational Operator2/2, Relational Operator1/2
  Saturation_S16/2 -> Terminator1/1
  Logical Operator1/1 -> Switch8/2
  CrCtl_trqIWinOld_mp/1 -> Switch8/1
  Switch8/1 -> CrCtl_trqReqIWin_mp/1

== system CrCtl_Governor/Resume From Below/CRCTL_SUBPRECRUISE/CrCtl_Suspend ==
  PT_trqWhlMinEng : Inport
  CrCtl_trqReqOld : Inport  Port=2
  AccPed_trqDes : Inport  Port=3
  CrCtl_trqLimAct : Inport  Port=4
  CrCtl_stSuspAct : Inport  Port=5
  Constant : Constant  Value=true
  Constant1 : Constant  Value=CrCtl_stSuspRamp_conv.CRCTL_SUSPENDENDRAMP
  Constant2 : Constant  Value=CrCtl_stSuspRamp_conv.CRCTL_SUSPENDRAMPDONE
  Constant3 : Constant  Value=CrCtl_stSuspRamp_conv.CRCTL_SUSPENDNOTACTIVE
  Constant4 : Constant  Value=CrCtl_stSuspRamp_conv.CRCTL_SUSPENDSTARTRAMP
  EdgeFalling : CXLib/EdgeFalling
  EdgeRising : CXLib/EdgeRising
  EdgeRising1 : CXLib/EdgeRising
  Logical Operator : Logic  Operator=NOT  AllPortsSameDT=off  OutDataTypeStr=boolean
  Subsystem : Subsystem
  Subsystem1 : Subsystem
  Switch{,1..3,5} (5 alike) : Switch  Criteria=u2 ~= 0
  Unit Delay : UnitDelay  SampleTime=-1
  CrCtl_stSuspRamp : Outport
  " CrCtl_trqReq" : Outport  Port=2
  wires:
  Subsystem/1(Out) -> Switch1/2, Subsystem1/5(In1)
  Subsystem/2(Out1) -> Switch5/1, Subsystem1/6(In2)
  PT_trqWhlMinEng/1 -> Subsystem/1(PT_trqWhlMinEng), Subsystem1/1(PT_trqWhlMinEng)
  CrCtl_trqReqOld/1 -> Subsystem/2(CrCtl_trqReqOld), Subsystem1/2(CrCtl_trqReqOld)
  CrCtl_trqLimAct/1 -> Subsystem1/4(CrCtl_trqLimAct)
  AccPed_trqDes/1 -> Subsystem1/3(AccPed_trqDes)
  Switch1/1 -> Switch/1
  Switch2/1 -> Switch/3
  Constant4/1 -> Switch1/1
  Constant2/1 -> Switch1/3
  Constant1/1 -> Switch2/1
  Constant3/1 -> Switch2/3
  Switch/1 -> CrCtl_stSuspRamp/1
  Subsystem1/1(Out1) -> Switch2/2
  Switch5/1 -> " CrCtl_trqReq"/1
  Subsystem1/2(Out2) -> Switch5/3
  Logical Operator/1 -> EdgeRising1/1
  EdgeRising/1 -> Subsystem/3(CrCtl_stSuspAct)
  EdgeRising1/1 -> Subsystem1/7(In3)
  CrCtl_stSuspAct/1 -> EdgeRising/1, EdgeFalling/1, Logical Operator/1, Subsystem/Enable, Switch/2, Switch5/2
  Constant/1 -> Switch3/1
  EdgeFalling/1 -> Switch3/2
  Switch3/1 -> Unit Delay/1, Subsystem1/Enable
  Unit Delay/1 -> Switch3/3

== system CrCtl_Governor/Resume From Below/CRCTL_SUBPRECRUISE/Governor ==
  CrCtl_trqLimAct : Inport
  CrCtl_trqMin : Inport  Port=2
  CrCtl_stGearRng_mp : Inport  Port=3
  CrCtl_vDesAct : Inport  Port=4
  stvHysEngBrkReq : Inport  Port=5
  GlbDa_vXFlt : Inport  Port=6
  stCrCtlOn : Inport  Port=7
  In1 : Inport  Port=8
  In2 : Inport  Port=9
  Enable : EnablePort
  Add1 : Sum  Inputs=+-
  Add2 : Sum  OutDataTypeStr=Trq_Nm
  Add3 : Sum  AccumDataTypeStr=Trq_Nm
  Constant : Constant  Value=CrCtl_swtILimWithP_C
  Constant1 : Constant  Value=CrCtl_Governor_DT
  Constant2 : Constant  Value=1000  OutDataTypeStr=Inherit: Inherit via back propagation
  CrCtl_ARW : Subsystem
  I_S16 : CXLib/I_S16
  PT1 Filtered Torque : Subsystem
  P_S16 : CXLib/P_S16
  Parameter Selection for Ki : Subsystem
  Parameter Selection for Kp : Subsystem
  Product : Product  OutDataTypeStr=uint32
  Saturation_S16 : CXLib/Saturation_S16
  Switch : Switch  Criteria=u2 ~= 0
  Terminator : Terminator
  Unit Delay : UnitDelay  SampleTime=-1
  Unit Delay1 : UnitDelay  SampleTime=-1
  CrCtl_trqReq : Outport
  CrCtl_trqIWinOld_mp : Outport  Port=2  OutDataTypeStr=Trq_Nm
  CrCtl_trqReqPWin_mp : Outport  Port=3
  wires:
  CrCtl_vDesAct/1 -> Add1/1
  GlbDa_vXFlt/1 -> Add1/2
  Add1/1 -> PT1 Filtered Torque/2(vDiffCrCtl), I_S16/1, P_S16/1
  Add2/1 -> Add3/1
  PT1 Filtered Torque/1(CrCtl_trqDesvHys) -> Add3/2
  Add3/1 -> Saturation_S16/1
  CrCtl_trqMin/1 -> CrCtl_ARW/2(CrCtl_trqMin), Saturation_S16/2
  CrCtl_trqLimAct/1 -> CrCtl_ARW/3(CrCtl_trqLimAct), Saturation_S16/3
  Saturation_S16/2 -> Terminator/1
  Saturation_S16/1 -> CrCtl_trqReq/1
  Switch/1 -> Add2/2, CrCtl_ARW/5(CrCtl_trqReqIWin_mp), CrCtl_trqIWinOld_mp/1
  Constant/1 -> CrCtl_ARW/1(CrCtl_swtILimWithP_C)
  stvHysEngBrkReq/1 -> PT1 Filtered Torque/1(stvHysEngBrkReq)
  CrCtl_stGearRng_mp/1 -> Parameter Selection for Kp/1(CrCtl_stGearRng_mp), Parameter Selection for Ki/1(CrCtl_stGearRng_mp), PT1 Filtered Torque/3(CrCtl_stGearRng_mp)
  stCrCtlOn/1 -> PT1 Filtered Torque/4(stCrCtlOn)
  Parameter Selection for Kp/1(Out1) -> P_S16/2
  Parameter Selection for Kp/2(Out2) -> P_S16/3
  Parameter Selection for Kp/3(Out3) -> P_S16/4
  Parameter Selection for Kp/4(Out4) -> P_S16/5
  Parameter Selection for Kp/5(Out5) -> P_S16/6
  Parameter Selection for Ki/1(Out1) -> I_S16/3
  Parameter Selection for Ki/2(Out2) -> I_S16/4
  Parameter Selection for Ki/3(Out3) -> I_S16/5
  Parameter Selection for Ki/4(Out4) -> I_S16/6
  Parameter Selection for Ki/5(Out5) -> I_S16/7
  CrCtl_ARW/2(Limit) -> Unit Delay1/1
  CrCtl_ARW/1(CrCtl_stInit_mp) -> Unit Delay/1
  Product/1 -> I_S16/2
  Constant2/1 -> Product/2
  Constant1/1 -> Product/1
  P_S16/1 -> CrCtl_trqReqPWin_mp/1, CrCtl_ARW/4(CrCtl_trqReqPWin_mp), Add2/1
  In1/1 -> I_S16/8
  In2/1 -> I_S16/9
  I_S16/1 -> Switch/3
  Unit Delay/1 -> Switch/2
  Unit Delay1/1 -> Switch/1

== system CrCtl_Governor/Resume From Below/CRCTL_SUBRMP/CrCtl_OverRide ==
  CrCtl_trqLimAct : Inport
  CrCtl_trqMin : Inport  Port=2
  APP_r : Inport  Port=3
  AccPed_trqDes : Inport  Port=4
  CrCtl_vDes : Inport  Port=5
  GlbDa_vXFlt : Inport  Port=6
  CrCtl_trqReq : Inport  Port=7
  CrCtl_trqIWinOld_mp : Inport  Port=8
  Add : Sum
  Bit Clear : simulink/Logic and Bit Operations/Bit Clear  iBit=1
  Bit Clear7 : simulink/Logic and Bit Operations/Bit Clear  iBit=0
  Bit Set : simulink/Logic and Bit Operations/Bit Set  iBit=1
  Bit Set7 : simulink/Logic and Bit Operations/Bit Set  iBit=0
  Constant : Constant  Value=0
  Constant2 : Constant  Value=CrCtl_vCnclOverride_C
  Constant8 : Constant  Value=CrCtl_swtOvrRdeFrzInteg_C
  Logical Operator : Logic  AllPortsSameDT=off  OutDataTypeStr=boolean
  Logical Operator1 : Logic  AllPortsSameDT=off  OutDataTypeStr=boolean
  Relational Operator : RelationalOperator  Operator=>  OutDataTypeStr=boolean  RndMeth=Simplest
  Relational Operator1 : RelationalOperator  Operator=>  OutDataTypeStr=boolean  RndMeth=Simplest
  Relational Operator2 : RelationalOperator  Operator=<=  OutDataTypeStr=boolean  RndMeth=Simplest
  Relational Operator3 : RelationalOperator  Operator=<  OutDataTypeStr=boolean  RndMeth=Simplest
  Saturation_S16 : CXLib/Saturation_S16
  Switch : Switch  Criteria=u2 ~= 0
  Switch7 : Switch  Criteria=u2 ~= 0
  Switch8 : Switch  Criteria=u2 ~= 0
  Terminator1 : Terminator
  Unit Delay : UnitDelay  SampleTime=-1
  CrCtl_stIWin_mp : Outport
  CrCtl_trqReqIWin_mp : Outport  Port=2
  wires:
  APP_r/1 -> Relational Operator/1
  Constant/1 -> Relational Operator/2
  AccPed_trqDes/1 -> Relational Operator1/1, Relational Operator2/1
  Relational Operator/1 -> Logical Operator/1
  Relational Operator1/1 -> Logical Operator/2
  Logical Operator/1 -> Switch/2
  Relational Operator2/1 -> Logical Operator1/1
  Relational Operator3/1 -> Logical Operator1/2
  GlbDa_vXFlt/1 -> Relational Operator3/1
  CrCtl_vDes/1 -> Add/1
  Add/1 -> Relational Operator3/2
  Constant2/1 -> Add/2
  CrCtl_trqLimAct/1 -> Saturation_S16/3
  CrCtl_trqMin/1 -> Saturation_S16/2
  Bit Set/1 -> Switch/1
  Bit Clear/1 -> Switch/3
  Switch/1 -> Bit Clear7/1, Bit Set7/1
  Constant8/1 -> Switch7/2
  Bit Set7/1 -> Switch7/1
  Bit Clear7/1 -> Switch7/3
  Switch7/1 -> CrCtl_stIWin_mp/1, Unit Delay/1
  Unit Delay/1 -> Bit Set/1, Bit Clear/1
  CrCtl_trqReq/1 -> Saturation_S16/1
  Saturation_S16/1 -> Switch8/3, Relational Operator2/2, Relational Operator1/2
  Saturation_S16/2 -> Terminator1/1
  Logical Operator1/1 -> Switch8/2
  CrCtl_trqIWinOld_mp/1 -> Switch8/1
  Switch8/1 -> CrCtl_trqReqIWin_mp/1

== system CrCtl_Governor/Resume From Below/CRCTL_SUBRMP/CrCtl_Suspend ==
  PT_trqWhlMinEng : Inport
  CrCtl_trqReqOld : Inport  Port=2
  AccPed_trqDes : Inport  Port=3
  CrCtl_trqLimAct : Inport  Port=4
  CrCtl_stSuspAct : Inport  Port=5
  Constant : Constant  Value=true
  Constant1 : Constant  Value=CrCtl_stSuspRamp_conv.CRCTL_SUSPENDENDRAMP
  Constant2 : Constant  Value=CrCtl_stSuspRamp_conv.CRCTL_SUSPENDRAMPDONE
  Constant3 : Constant  Value=CrCtl_stSuspRamp_conv.CRCTL_SUSPENDNOTACTIVE
  Constant4 : Constant  Value=CrCtl_stSuspRamp_conv.CRCTL_SUSPENDSTARTRAMP
  EdgeFalling : CXLib/EdgeFalling
  EdgeRising : CXLib/EdgeRising
  EdgeRising1 : CXLib/EdgeRising
  Logical Operator : Logic  Operator=NOT  AllPortsSameDT=off  OutDataTypeStr=boolean
  Subsystem : Subsystem
  Subsystem1 : Subsystem
  Switch{,1..3,5} (5 alike) : Switch  Criteria=u2 ~= 0
  Unit Delay : UnitDelay  SampleTime=-1
  CrCtl_stSuspRamp : Outport
  " CrCtl_trqReq" : Outport  Port=2
  wires:
  Subsystem/1(Out) -> Switch1/2, Subsystem1/5(In1)
  Subsystem/2(Out1) -> Switch5/1, Subsystem1/6(In2)
  PT_trqWhlMinEng/1 -> Subsystem/1(PT_trqWhlMinEng), Subsystem1/1(PT_trqWhlMinEng)
  CrCtl_trqReqOld/1 -> Subsystem/2(CrCtl_trqReqOld), Subsystem1/2(CrCtl_trqReqOld)
  CrCtl_trqLimAct/1 -> Subsystem1/4(CrCtl_trqLimAct)
  AccPed_trqDes/1 -> Subsystem1/3(AccPed_trqDes)
  Switch1/1 -> Switch/1
  Switch2/1 -> Switch/3
  Constant4/1 -> Switch1/1
  Constant2/1 -> Switch1/3
  Constant1/1 -> Switch2/1
  Constant3/1 -> Switch2/3
  Switch/1 -> CrCtl_stSuspRamp/1
  Subsystem1/1(Out1) -> Switch2/2
  Switch5/1 -> " CrCtl_trqReq"/1
  Subsystem1/2(Out2) -> Switch5/3
  Logical Operator/1 -> EdgeRising1/1
  EdgeRising/1 -> Subsystem/3(CrCtl_stSuspAct)
  EdgeRising1/1 -> Subsystem1/7(In3)
  CrCtl_stSuspAct/1 -> EdgeRising/1, EdgeFalling/1, Logical Operator/1, Subsystem/Enable, Switch/2, Switch5/2
  Constant/1 -> Switch3/1
  EdgeFalling/1 -> Switch3/2
  Switch3/1 -> Unit Delay/1, Subsystem1/Enable
  Unit Delay/1 -> Switch3/3
